simulink library "DoubletsLib"  (R2024b)
settings: Solver=VariableStepAuto  StartTime=0.0  StopTime=10.0  RelTol=1e-3
undefined symbols (not defined in the file): SimPar
libraries: simulink x15
settings Model: Creator=tbritton  LastModifiedBy=gryph
settings SolverCC: AlgebraicLoopSolver=TrustRegion
settings OptimizationCC: ReuseModelBlockBuffer=off
settings DebuggingCC: UnconnectedInputMsg=warning  UnconnectedOutputMsg=warning  UnconnectedLineMsg=warning
settings ModelReferenceCC: EnableRefExpFcnMdlSchedulingChecks=on
settings RTWCC: GPUComputeCapability=3.5  DLArmComputeVersion=19.05

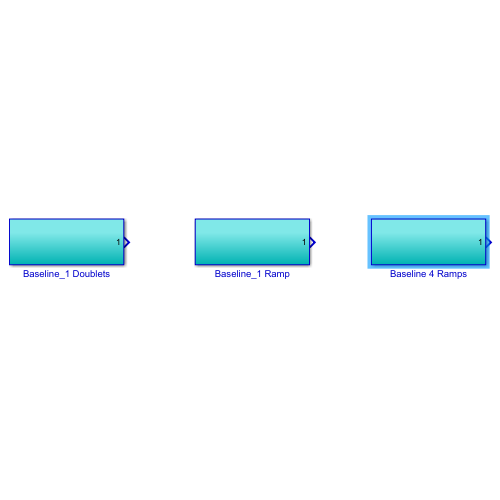
[thumbnail: Simulink's stored preview of the top-level diagram]
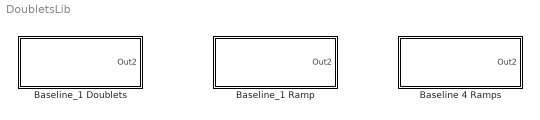
== system DoubletsLib ==
  Baseline 4 Ramps : Subsystem
  Baseline_1 Doublets : Subsystem
  Baseline_1 Ramp : Subsystem

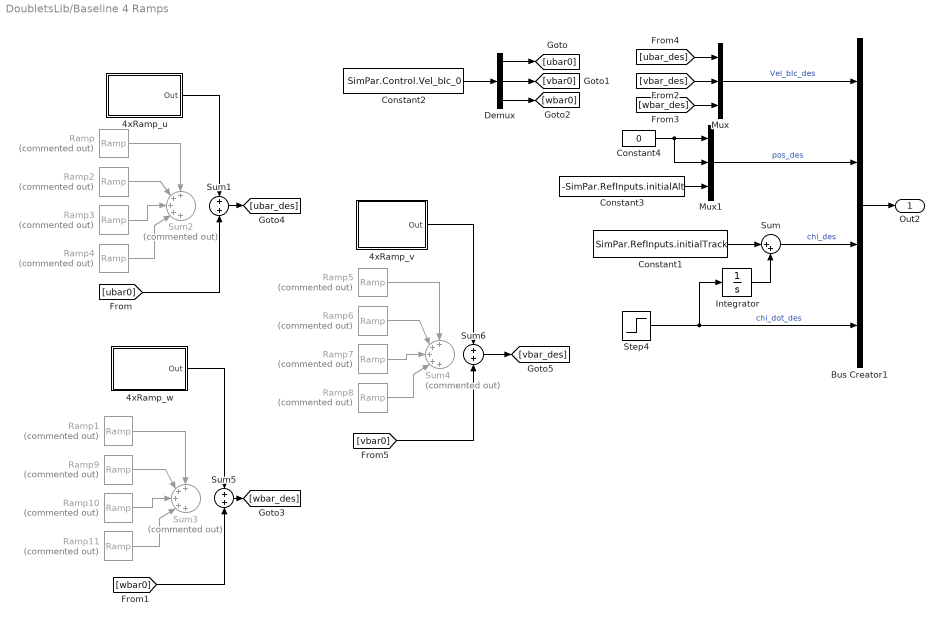
== system DoubletsLib/Baseline 4 Ramps ==
  4xRamp_u : Subsystem  mask{InitialOutput=[SimPar.RefInputs.ramps.Vel_initialValue1(1); SimPar.RefInputs.ramps.Vel_initialValue2(1); SimPar.RefInputs.ramps.Vel_initialValue3(1); SimPar.RefInputs.ramps.Vel_initialValue4(1)], start=[SimPar.RefInputs.ramps.Vel_startTime1(1); SimPar.RefInputs.ramps.Vel_startTime2(1); SimPar.RefInputs.ramps.Vel_startTime3(1); SimPar.RefInputs.ramps.Vel_startTime4(1)], slope=[SimPar.RefInputs.ramps.Vel_slope1(1); SimPar.RefInputs.ramps.Vel_slope2(1); SimPar.RefInputs.ramps.Vel_slope3(1); SimPar.RefInputs.ramps.Vel_slope4(1)]}
      mask prompts: InitialOutput "Initial Conditions"; start "Starting times for ramps"; slope "Slopes of ramps"
      mask help:
      | Generates a series of 4 ramps.
      | Inputs must be provided as vectors of 4 elements.
  4xRamp_v : Subsystem  mask{InitialOutput=[SimPar.RefInputs.ramps.Vel_initialValue1(2); SimPar.RefInputs.ramps.Vel_initialValue2(2); SimPar.RefInputs.ramps.Vel_initialValue3(2); SimPar.RefInputs.ramps.Vel_initialValue4(2)], start=[SimPar.RefInputs.ramps.Vel_startTime1(2); SimPar.RefInputs.ramps.Vel_startTime2(2); SimPar.RefInputs.ramps.Vel_startTime3(2); SimPar.RefInputs.ramps.Vel_startTime4(2)], slope=[SimPar.RefInputs.ramps.Vel_slope1(2); SimPar.RefInputs.ramps.Vel_slope2(2); SimPar.RefInputs.ramps.Vel_slope3(2); SimPar.RefInputs.ramps.Vel_slope4(2)]}
      mask prompts: InitialOutput "Initial Conditions"; start "Starting times for ramps"; slope "Slopes of ramps"
      mask help:
      | Generates a series of 4 ramps.
      | Inputs must be provided as vectors of 4 elements.
  4xRamp_w : Subsystem  mask{InitialOutput=[SimPar.RefInputs.ramps.Vel_initialValue1(3); SimPar.RefInputs.ramps.Vel_initialValue2(3); SimPar.RefInputs.ramps.Vel_initialValue3(3); SimPar.RefInputs.ramps.Vel_initialValue4(3)], start=[SimPar.RefInputs.ramps.Vel_startTime1(3); SimPar.RefInputs.ramps.Vel_startTime2(3); SimPar.RefInputs.ramps.Vel_startTime3(3); SimPar.RefInputs.ramps.Vel_startTime4(3)], slope=[SimPar.RefInputs.ramps.Vel_slope1(3); SimPar.RefInputs.ramps.Vel_slope2(3); SimPar.RefInputs.ramps.Vel_slope3(3); SimPar.RefInputs.ramps.Vel_slope4(3)]}
      mask prompts: InitialOutput "Initial Conditions"; start "Starting times for ramps"; slope "Slopes of ramps"
      mask help:
      | Generates a series of 4 ramps.
      | Inputs must be provided as vectors of 4 elements.
  Bus Creator1 : BusCreator  Inputs=4  OutDataTypeStr=Bus: BUS_REF_INPUT
  Constant1 : Constant  Value=SimPar.RefInputs.initialTrack
  Constant2 : Constant  Value=SimPar.Control.Vel_bIc_0
  Constant3 : Constant  Value=-SimPar.RefInputs.initialAlt
  Constant4 : Constant  Value=0
  Demux : Demux  Outputs=3
  Integrator : Integrator
  Mux : Mux  Inputs=3
  Mux1 : Mux  Inputs=3
  Ramp : simulink/Sources/Ramp  Commented=on  slope=SimPar.RefInputs.ramps.Vel_slope1(1)  start=SimPar.RefInputs.ramps.Vel_startTime1(1)  InitialOutput=SimPar.RefInputs.ramps.Vel_initialValue1(1)
  Ramp1 : simulink/Sources/Ramp  Commented=on  slope=SimPar.RefInputs.ramps.Vel_slope1(3)  start=SimPar.RefInputs.ramps.Vel_startTime1(3)  InitialOutput=SimPar.RefInputs.ramps.Vel_initialValue1(3)
  Ramp10 : simulink/Sources/Ramp  Commented=on  slope=SimPar.RefInputs.ramps.Vel_slope3(3)  start=SimPar.RefInputs.ramps.Vel_startTime3(3)  InitialOutput=SimPar.RefInputs.ramps.Vel_initialValue3(3)
  Ramp11 : simulink/Sources/Ramp  Commented=on  slope=SimPar.RefInputs.ramps.Vel_slope4(3)  start=SimPar.RefInputs.ramps.Vel_startTime4(3)  InitialOutput=SimPar.RefInputs.ramps.Vel_initialValue4(3)
  Ramp2 : simulink/Sources/Ramp  Commented=on  slope=SimPar.RefInputs.ramps.Vel_slope2(1)  start=SimPar.RefInputs.ramps.Vel_startTime2(1)  InitialOutput=SimPar.RefInputs.ramps.Vel_initialValue2(1)
  Ramp3 : simulink/Sources/Ramp  Commented=on  slope=SimPar.RefInputs.ramps.Vel_slope3(1)  start=SimPar.RefInputs.ramps.Vel_startTime3(1)  InitialOutput=SimPar.RefInputs.ramps.Vel_initialValue3(1)
  Ramp4 : simulink/Sources/Ramp  Commented=on  slope=SimPar.RefInputs.ramps.Vel_slope4(1)  start=SimPar.RefInputs.ramps.Vel_startTime4(1)  InitialOutput=SimPar.RefInputs.ramps.Vel_initialValue4(1)
  Ramp5 : simulink/Sources/Ramp  Commented=on  slope=SimPar.RefInputs.ramps.Vel_slope1(2)  start=SimPar.RefInputs.ramps.Vel_startTime1(2)  InitialOutput=SimPar.RefInputs.ramps.Vel_initialValue1(2)
  Ramp6 : simulink/Sources/Ramp  Commented=on  slope=SimPar.RefInputs.ramps.Vel_slope2(2)  start=SimPar.RefInputs.ramps.Vel_startTime2(2)  InitialOutput=SimPar.RefInputs.ramps.Vel_initialValue2(2)
  Ramp7 : simulink/Sources/Ramp  Commented=on  slope=SimPar.RefInputs.ramps.Vel_slope3(2)  start=SimPar.RefInputs.ramps.Vel_startTime3(2)  InitialOutput=SimPar.RefInputs.ramps.Vel_initialValue3(2)
  Ramp8 : simulink/Sources/Ramp  Commented=on  slope=SimPar.RefInputs.ramps.Vel_slope4(2)  start=SimPar.RefInputs.ramps.Vel_startTime4(2)  InitialOutput=SimPar.RefInputs.ramps.Vel_initialValue4(2)
  Ramp9 : simulink/Sources/Ramp  Commented=on  slope=SimPar.RefInputs.ramps.Vel_slope2(3)  start=SimPar.RefInputs.ramps.Vel_startTime2(3)  InitialOutput=SimPar.RefInputs.ramps.Vel_initialValue2(3)
  Step4 : Step  Time=SimPar.RefInputs.doublets.Track_stepTime  Before=SimPar.RefInputs.doublets.Track_initialValue  After=SimPar.RefInputs.doublets.Track_finalValue  SampleTime=0
  Sum : Sum  Inputs=|++
  Sum1 : Sum  Inputs=+|+
  Sum2 : Sum  Commented=on  Inputs=+++++
  Sum3 : Sum  Commented=on  Inputs=+++++
  Sum4 : Sum  Commented=on  Inputs=+++++
  Sum5 : Sum  Inputs=+|+
  Sum6 : Sum  Inputs=+|+
  Out2 : Outport
  wires:
  Constant4/1 -> Mux1/2, Mux1/1
  Constant3/1 -> Mux1/3
  Ramp/1 -> Sum2/1
  Integrator/1 -> Sum/2
  Sum/1 -> Bus Creator1/3  "chi_des"
  [ubar_des] -> Mux/1
  [wbar_des] -> Mux/3
  Constant1/1 -> Sum/1
  Step4/1 -> Bus Creator1/4, Integrator/1  "chi_dot_des"
  [vbar_des] -> Mux/2
  [ubar0] -> Sum1/2
  Bus Creator1/1 -> Out2/1
  Mux/1 -> Bus Creator1/1  "Vel_bIc_des"
  Mux1/1 -> Bus Creator1/2  "pos_des"
  Demux/1 -> [ubar0]
  Demux/3 -> [wbar0]
  Demux/2 -> [vbar0]
  Constant2/1 -> Demux/1
  Ramp2/1 -> Sum2/2
  Ramp3/1 -> Sum2/3
  Ramp4/1 -> Sum2/4
  [vbar0] -> Sum6/2
  Ramp5/1 -> Sum4/1
  Ramp6/1 -> Sum4/2
  Ramp7/1 -> Sum4/3
  Ramp8/1 -> Sum4/4
  Ramp11/1 -> Sum3/4
  Ramp10/1 -> Sum3/3
  Ramp9/1 -> Sum3/2
  Ramp1/1 -> Sum3/1
  Sum1/1 -> [ubar_des]
  4xRamp_u/1(Out) -> Sum1/1
  Sum6/1 -> [vbar_des]
  [wbar0] -> Sum5/2
  Sum5/1 -> [wbar_des]
  4xRamp_w/1(Out) -> Sum5/1
  4xRamp_v/1(Out) -> Sum6/1

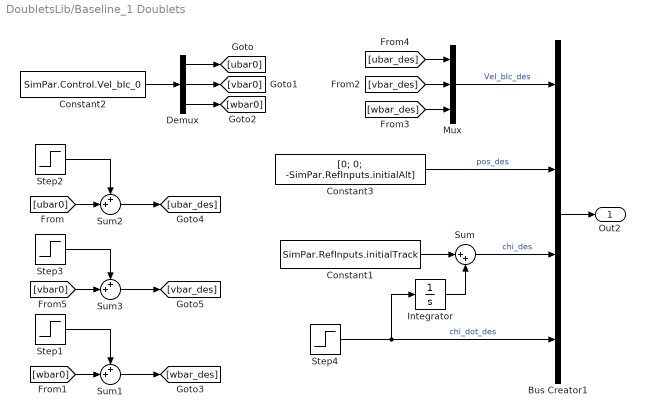
== system DoubletsLib/Baseline_1 Doublets ==
  Bus Creator1 : BusCreator  Inputs=4  OutDataTypeStr=Bus: BUS_REF_INPUT
  Constant1 : Constant  Value=SimPar.RefInputs.initialTrack
  Constant2 : Constant  Value=SimPar.Control.Vel_bIc_0
  Constant3 : Constant  Value=[0; 0; -SimPar.RefInputs.initialAlt]
  Demux : Demux  Outputs=3
  Integrator : Integrator
  Mux : Mux  Inputs=3
  Step1 : Step  Time=SimPar.RefInputs.doublets.Vel_stepTime(3)  Before=SimPar.RefInputs.doublets.Vel_initialValue(3)  After=SimPar.RefInputs.doublets.Vel_finalValue(3)  SampleTime=0
  Step2 : Step  Time=SimPar.RefInputs.doublets.Vel_stepTime(1)  Before=SimPar.RefInputs.doublets.Vel_initialValue(1)  After=SimPar.RefInputs.doublets.Vel_finalValue(1)  SampleTime=0
  Step3 : Step  Time=SimPar.RefInputs.doublets.Vel_stepTime(2)  Before=SimPar.RefInputs.doublets.Vel_initialValue(2)  After=SimPar.RefInputs.doublets.Vel_finalValue(2)  SampleTime=0
  Step4 : Step  Time=SimPar.RefInputs.doublets.Track_stepTime  Before=SimPar.RefInputs.doublets.Track_initialValue  After=SimPar.RefInputs.doublets.Track_finalValue  SampleTime=0
  Sum : Sum  Inputs=|++
  Sum1 : Sum  Inputs=++|
  Sum2 : Sum  Inputs=++|
  Sum3 : Sum  Inputs=++|
  Out2 : Outport
  wires:
  Constant2/1 -> Demux/1
  Demux/2 -> [vbar0]
  Demux/3 -> [wbar0]
  Sum1/1 -> [wbar_des]
  Demux/1 -> [ubar0]
  Constant3/1 -> Bus Creator1/2  "pos_des"
  Mux/1 -> Bus Creator1/1  "Vel_bIc_des"
  Bus Creator1/1 -> Out2/1
  [ubar0] -> Sum2/2
  [wbar0] -> Sum1/2
  [vbar_des] -> Mux/2
  Step4/1 -> Integrator/1, Bus Creator1/4  "chi_dot_des"
  Constant1/1 -> Sum/1
  [wbar_des] -> Mux/3
  [ubar_des] -> Mux/1
  Sum2/1 -> [ubar_des]
  [vbar0] -> Sum3/2
  Sum3/1 -> [vbar_des]
  Sum/1 -> Bus Creator1/3  "chi_des"
  Integrator/1 -> Sum/2
  Step1/1 -> Sum1/1
  Step3/1 -> Sum3/1
  Step2/1 -> Sum2/1

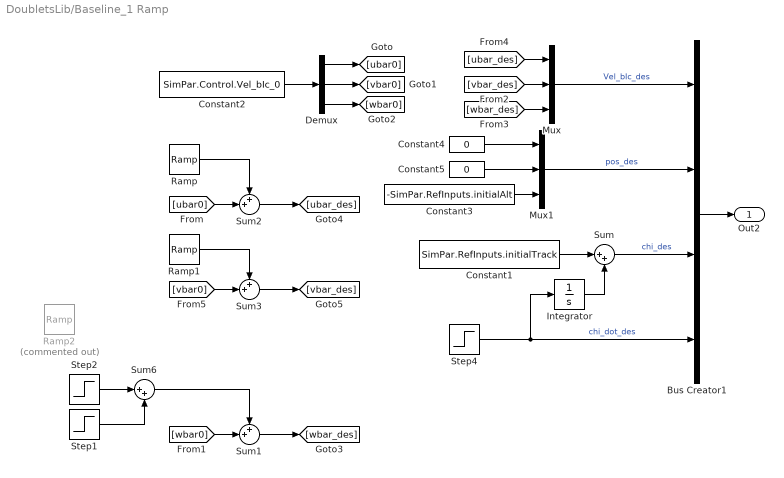
== system DoubletsLib/Baseline_1 Ramp ==
  Bus Creator1 : BusCreator  Inputs=4  OutDataTypeStr=Bus: BUS_REF_INPUT
  Constant1 : Constant  Value=SimPar.RefInputs.initialTrack
  Constant2 : Constant  Value=SimPar.Control.Vel_bIc_0
  Constant3 : Constant  Value=-SimPar.RefInputs.initialAlt
  Constant4 : Constant  Value=0
  Constant5 : Constant  Value=0
  Demux : Demux  Outputs=3
  Integrator : Integrator
  Mux : Mux  Inputs=3
  Mux1 : Mux  Inputs=3
  Ramp : simulink/Sources/Ramp  slope=SimPar.RefInputs.ramps.Vel_slope(1)  start=SimPar.RefInputs.ramps.Vel_startTime(1)  InitialOutput=SimPar.RefInputs.ramps.Vel_initialValue(1)
  Ramp1 : simulink/Sources/Ramp  slope=SimPar.RefInputs.ramps.Vel_slope(2)  start=SimPar.RefInputs.ramps.Vel_startTime(2)  InitialOutput=SimPar.RefInputs.ramps.Vel_initialValue(2)
  Ramp2 : simulink/Sources/Ramp  Commented=on  slope=SimPar.RefInputs.ramps.Vel_slope(3)  start=SimPar.RefInputs.ramps.Vel_startTime(3)  InitialOutput=SimPar.RefInputs.ramps.Vel_initialValue(3)
  Step1 : Step  Time=SimPar.RefInputs.doublets.Vel_stepTime(3)+50  Before=SimPar.RefInputs.doublets.Vel_initialValue(3)  After=-SimPar.RefInputs.doublets.Vel_finalValue(3)  SampleTime=0
  Step2 : Step  Time=SimPar.RefInputs.doublets.Vel_stepTime(3)  Before=SimPar.RefInputs.doublets.Vel_initialValue(3)  After=SimPar.RefInputs.doublets.Vel_finalValue(3)  SampleTime=0
  Step4 : Step  Time=SimPar.RefInputs.doublets.Track_stepTime  Before=SimPar.RefInputs.doublets.Track_initialValue  After=SimPar.RefInputs.doublets.Track_finalValue  SampleTime=0
  Sum : Sum  Inputs=|++
  Sum1 : Sum  Inputs=++|
  Sum2 : Sum  Inputs=++|
  Sum3 : Sum  Inputs=++|
  Sum6 : Sum  Inputs=|++
  Out2 : Outport
  wires:
  Constant2/1 -> Demux/1
  Demux/2 -> [vbar0]
  Demux/3 -> [wbar0]
  Sum1/1 -> [wbar_des]
  Demux/1 -> [ubar0]
  Mux1/1 -> Bus Creator1/2  "pos_des"
  Mux/1 -> Bus Creator1/1  "Vel_bIc_des"
  Bus Creator1/1 -> Out2/1
  [ubar0] -> Sum2/2
  [wbar0] -> Sum1/2
  [vbar_des] -> Mux/2
  Step4/1 -> Integrator/1, Bus Creator1/4  "chi_dot_des"
  Constant1/1 -> Sum/1
  [wbar_des] -> Mux/3
  [ubar_des] -> Mux/1
  Sum2/1 -> [ubar_des]
  [vbar0] -> Sum3/2
  Sum3/1 -> [vbar_des]
  Sum/1 -> Bus Creator1/3  "chi_des"
  Integrator/1 -> Sum/2
  Sum6/1 -> Sum1/1
  Ramp1/1 -> Sum3/1
  Ramp/1 -> Sum2/1
  Step2/1 -> Sum6/1
  Step1/1 -> Sum6/2
  Constant3/1 -> Mux1/3
  Constant4/1 -> Mux1/1
  Constant5/1 -> Mux1/2

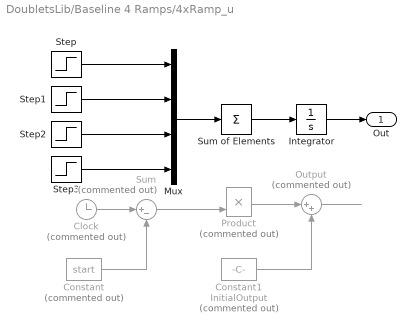
== system DoubletsLib/Baseline 4 Ramps/4xRamp_u ==
  Clock : Clock  Commented=on
      settings: DisableCoverage=on
  Constant : Constant  Commented=on  DisableCoverage=on  Value=start  OutDataTypeStr=Inherit: Inherit via back propagation
  Constant1 : Constant  Commented=on  DisableCoverage=on  Value=InitialOutput  OutDataTypeStr=Inherit: Inherit via back propagation
  Integrator : Integrator  InitialCondition=sum(InitialOutput)
  Mux : Mux
  Output : Sum  Commented=on  Inputs=|++  InputSameDT=on  SaturateOnIntegerOverflow=on  OutDataTypeStr=Inherit: Same as first input
  Product : Product  Commented=on  DisableCoverage=on  InputSameDT=on  SaturateOnIntegerOverflow=on  OutDataTypeStr=Inherit: Same as first input
  Step : Step  DisableCoverage=on  Time=start(1)  After=slope(1)  OutDataTypeStr=fixdt('double', 'DataTypeOverride', 'Off')  SampleTime=0
  Step1 : Step  DisableCoverage=on  Time=start(2)  After=slope(2)  OutDataTypeStr=fixdt('double', 'DataTypeOverride', 'Off')  SampleTime=0
  Step2 : Step  DisableCoverage=on  Time=start(3)  After=slope(3)  OutDataTypeStr=fixdt('double', 'DataTypeOverride', 'Off')  SampleTime=0
  Step3 : Step  DisableCoverage=on  Time=start(4)  After=slope(4)  OutDataTypeStr=fixdt('double', 'DataTypeOverride', 'Off')  SampleTime=0
  Sum : Sum  Commented=on  DisableCoverage=on  Inputs=|+-  InputSameDT=on  SaturateOnIntegerOverflow=on  OutDataTypeStr=Inherit: Same as first input
  Sum of Elements : Sum  Inputs=+
  Out : Outport
  wires:
  Output/1 -> ?
  Clock/1 -> Sum/1
  Constant1/1 -> Output/2
  Product/1 -> Output/1
  Sum/1 -> Product/2
  Constant/1 -> Sum/2
  Sum of Elements/1 -> Integrator/1
  Step/1 -> Mux/1
  Step1/1 -> Mux/2
  Step2/1 -> Mux/3
  Step3/1 -> Mux/4
  Mux/1 -> Sum of Elements/1
  Integrator/1 -> Out/1

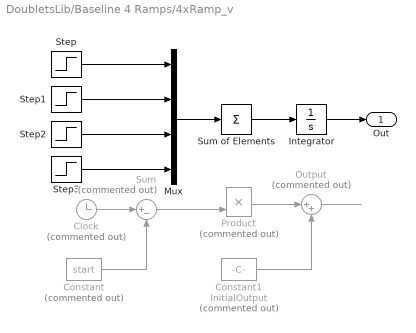
== system DoubletsLib/Baseline 4 Ramps/4xRamp_v ==
  Clock : Clock  Commented=on
      settings: DisableCoverage=on
  Constant : Constant  Commented=on  DisableCoverage=on  Value=start  OutDataTypeStr=Inherit: Inherit via back propagation
  Constant1 : Constant  Commented=on  DisableCoverage=on  Value=InitialOutput  OutDataTypeStr=Inherit: Inherit via back propagation
  Integrator : Integrator  InitialCondition=sum(InitialOutput)
  Mux : Mux
  Output : Sum  Commented=on  Inputs=|++  InputSameDT=on  SaturateOnIntegerOverflow=on  OutDataTypeStr=Inherit: Same as first input
  Product : Product  Commented=on  DisableCoverage=on  InputSameDT=on  SaturateOnIntegerOverflow=on  OutDataTypeStr=Inherit: Same as first input
  Step : Step  DisableCoverage=on  Time=start(1)  After=slope(1)  OutDataTypeStr=fixdt('double', 'DataTypeOverride', 'Off')  SampleTime=0
  Step1 : Step  DisableCoverage=on  Time=start(2)  After=slope(2)  OutDataTypeStr=fixdt('double', 'DataTypeOverride', 'Off')  SampleTime=0
  Step2 : Step  DisableCoverage=on  Time=start(3)  After=slope(3)  OutDataTypeStr=fixdt('double', 'DataTypeOverride', 'Off')  SampleTime=0
  Step3 : Step  DisableCoverage=on  Time=start(4)  After=slope(4)  OutDataTypeStr=fixdt('double', 'DataTypeOverride', 'Off')  SampleTime=0
  Sum : Sum  Commented=on  DisableCoverage=on  Inputs=|+-  InputSameDT=on  SaturateOnIntegerOverflow=on  OutDataTypeStr=Inherit: Same as first input
  Sum of Elements : Sum  Inputs=+
  Out : Outport
  wires:
  Integrator/1 -> Out/1
  Mux/1 -> Sum of Elements/1
  Step3/1 -> Mux/4
  Step2/1 -> Mux/3
  Step1/1 -> Mux/2
  Step/1 -> Mux/1
  Sum of Elements/1 -> Integrator/1
  Constant/1 -> Sum/2
  Sum/1 -> Product/2
  Product/1 -> Output/1
  Constant1/1 -> Output/2
  Clock/1 -> Sum/1
  Output/1 -> ?

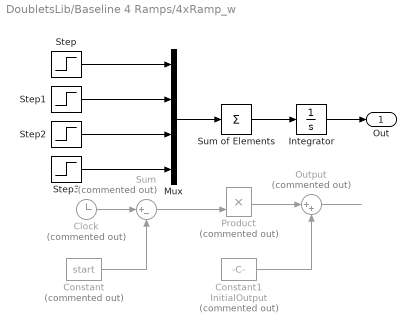
== system DoubletsLib/Baseline 4 Ramps/4xRamp_w ==
  Clock : Clock  Commented=on
      settings: DisableCoverage=on
  Constant : Constant  Commented=on  DisableCoverage=on  Value=start  OutDataTypeStr=Inherit: Inherit via back propagation
  Constant1 : Constant  Commented=on  DisableCoverage=on  Value=InitialOutput  OutDataTypeStr=Inherit: Inherit via back propagation
  Integrator : Integrator  InitialCondition=sum(InitialOutput)
  Mux : Mux
  Output : Sum  Commented=on  Inputs=|++  InputSameDT=on  SaturateOnIntegerOverflow=on  OutDataTypeStr=Inherit: Same as first input
  Product : Product  Commented=on  DisableCoverage=on  InputSameDT=on  SaturateOnIntegerOverflow=on  OutDataTypeStr=Inherit: Same as first input
  Step : Step  DisableCoverage=on  Time=start(1)  After=slope(1)  OutDataTypeStr=fixdt('double', 'DataTypeOverride', 'Off')  SampleTime=0
  Step1 : Step  DisableCoverage=on  Time=start(2)  After=slope(2)  OutDataTypeStr=fixdt('double', 'DataTypeOverride', 'Off')  SampleTime=0
  Step2 : Step  DisableCoverage=on  Time=start(3)  After=slope(3)  OutDataTypeStr=fixdt('double', 'DataTypeOverride', 'Off')  SampleTime=0
  Step3 : Step  DisableCoverage=on  Time=start(4)  After=slope(4)  OutDataTypeStr=fixdt('double', 'DataTypeOverride', 'Off')  SampleTime=0
  Sum : Sum  Commented=on  DisableCoverage=on  Inputs=|+-  InputSameDT=on  SaturateOnIntegerOverflow=on  OutDataTypeStr=Inherit: Same as first input
  Sum of Elements : Sum  Inputs=+
  Out : Outport
  wires:
  Output/1 -> ?
  Clock/1 -> Sum/1
  Constant1/1 -> Output/2
  Product/1 -> Output/1
  Sum/1 -> Product/2
  Constant/1 -> Sum/2
  Sum of Elements/1 -> Integrator/1
  Step/1 -> Mux/1
  Step1/1 -> Mux/2
  Step2/1 -> Mux/3
  Step3/1 -> Mux/4
  Mux/1 -> Sum of Elements/1
  Integrator/1 -> Out/1
